simulink model "powertrain"  (R2020b)
settings: Solver=FixedStepAuto  StartTime=0.0  StopTime=t(end)  RelTol=1e-3
PreLoadFcn:
  | C_sc = 1;
StartFcn:
  | C_sc = 1;
values from neighbouring files (symbols this model uses):
  D = 0    [model_fc.m]
  Ts = old_data.Ts    [model_fc.m]
undefined symbols (not defined in the file or in its folder): ANFIS, command, DiscIntNeverNeededParam, ECMS, Flight, in, Ion, Lithium, MPC, out, Tmpc, w
libraries: powerlib x25, neural x25, fuzblock x5, electricdrivelib x3, lib_converters x3, simulink x3, re_lib x1
(part 1 of 8)
PostSaveFcn:
  | C_sc = 1;
settings Model: SimulationMode=accelerator  Creator=maloc  LastModifiedBy=maloc
settings OptimizationCC: DefaultParameterBehavior=Inlined  EnhancedBackFolding=on  PassReuseOutputArgsAs=Individual arguments  ZeroExternalMemoryAtStartup=off  ZeroInternalMemoryAtStartup=off  OptimizeBlockOrder=speed  DifferentSizesBufferReuse=on  OptimizationCustomize=off  EfficientTunableParamExpr=on
settings DebuggingCC: ParameterTunabilityLossMsg=error  SFUnexpectedBacktrackingDiag=warning  SFNoUnconditionalDefaultTransitionDiag=warning
settings SFSimCC: MATLABDynamicMemAlloc=off
settings RTWCC: Description=Embedded Coder  SystemTargetFile=ert.tlc  GenCodeOnly=on  TemplateMakefile=ert_default_tmf  GenerateReport=on  BuildConfiguration=Debug  LaunchReport=on
settings CodeAppCC: ForceParamTrailComments=on  IgnoreCustomStorageClasses=off  OperatorAnnotations=on  SimulinkDataObjDesc=on  SFDataObjDesc=on  InsertBlockDesc=on  EnableCustomComments=on
settings ERTTargetCC: TargetLangStandard=C99 (ISO)  GenerateSampleERTMain=on  InlinedParameterPlacement=NonHierarchical  ERTCustomFileTemplate=example_file_process.tlc

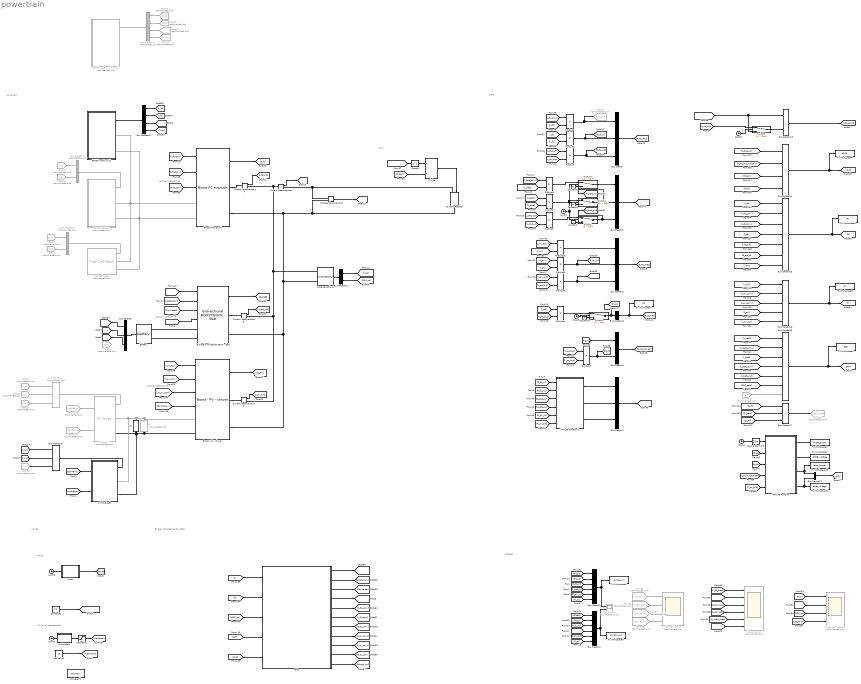
== system powertrain ==
  note: ACTIVE / DESACTIVE
  note: Pload
  note: Data
  note: Powertrain
  note: Energy Management System
  note: SCOPES
  note: Load
  note: Inputs
  note: ACTIVE / DESACTIVE
  note: ACTIVE / DESACTIVE
  note: PV Panel weather data
  Battery : electricdrivelib/Extra Sources/Battery  BatType=Lithium-Ion  ShowTempParam=off  ThermalPreset=no  ShowAgeParam=off  NomV=48  NomQ=15  SOC=80  Batt_Tr=20  PresetModel=on  MaxQ=15  MinV=36  FullV=55.8714  Dis_rate=6.5217  R=0.032  Normal_OP=13.5652  expZone="[51.8585     0.736957]"  current=[2 5 10 40]  Units=Time  Tci=20  NomT=20  T2=-30  MaxQ2=4.8  FullV2=7.1  Normal_OP2=5.655  expZone2="[6.58           1]"  Rca=0.6  ti=2000  Dp=0  Neq0=0  Tsim=Ts  Ta1=25  Qeol=5.4*0.9  Reol=0.013333*1.2  Char_age=[2.3478, 3]  Dis_age=[2.3478, 10]  N1=1500  N2=10500  N3=1000  N4=1400  Ta2=45  N5=950
  Bidirectional BOOST/BUCK - Batt : lib_converters/Bidirectional BOOST//BUCK - Batt  n_buck=0.9  Tr_buck=0.1  damp_buck=0.707  n_boost=0.9  Tr_boost=0.1  damp_boost=0.707  max_curr=[30 -4]  Co=1e-4  CL=C_sc  Li=1e-3  Ts=Ts
  Boost - PV - chsvar : lib_converters/Boost - PV - chsvar  n=0.9  Co=1e-4  CL=C_sc  Li=2e-3  damp=0.707  Tr=0.1  Ts=Ts
  Boost FC avg-swh : lib_converters/Boost FC avg-swh  conv_type=Average model  n=0.9  Co=1e-4  CL=C_sc  Li=2e-3  damp=0.707  Tr=1  Ts=Ts
      link override Discrete PI Controller3: Ts=Ts
  Bus Creator : BusCreator  Inputs=command,in,out
  Bus Creator{1,5,7,17} (4 alike) : BusCreator  Inputs=3
  Bus Creator11 : BusCreator  Inputs=1
  Bus Creator12 : BusCreator  Inputs=2
  Bus Creator13 : BusCreator  Inputs=2
  Bus Creator14 : BusCreator  Inputs=4
  Bus Creator15 : BusCreator  Inputs=7
  Bus Creator16 : BusCreator  Inputs=5
  Bus Creator18 : BusCreator  Inputs=7
  Bus Creator2 : BusCreator  Inputs=6
  Bus Creator3 : BusCreator  Inputs=6
  Bus Creator6 : BusCreator  Inputs=2
  Bus Selector : BusSelector  OutputSignals=SOC (%),Current (A),Voltage (V)
  Bus Selector1 : BusSelector  OutputSignals=Current I,SOC %
  Bus Selector2 : BusSelector  Commented=on  OutputSignals=V_PV,I_PV,Temperature (deg C)
  Bus Selector3 : BusSelector  Commented=on  OutputSignals=Voltage,Current
  Bus Selector4 : BusSelector  Commented=on  OutputSignals=Vout,Ifc
  Bus Selector5 : BusSelector  OutputSignals=V_PV,I_PV,Temperature (deg C)
  Bus Selector6 : BusSelector  OutputSignals=Vout,Ifc,E_act_d,limit
  Bus Selector7 : BusSelector  Commented=on  OutputSignals=Vout,Ifc,E_act_d,limit
  C2 : powerlib/Elements/Series RLC Branch  LConnTagsString=__new0  RConnTagsString=__new0  BranchType=C  Resistance=0.01  Inductance=1e-3  SetiL0=off  InitialCurrent=0  Capacitance=1e-3  Setx0=off  InitialVoltage=0  Measurements=None
  Clock{1..6} (6 alike) : Clock
  Comparison : Scope  Commented=on  NumInputPorts=2
  Constant{,1..3} (4 alike) : Constant  Value=0
  Constant5 : Constant  Value=25
  Constant6 : Constant  Value=72
  Control output : Scope  Commented=on  NumInputPorts=4
  Current Measurement{,2..4} (4 alike) : powerlib/Measurements/Current Measurement  PhasorSimulation=off  OutputType=Complex  PSBequivalent=0
  Divide : Product  Inputs=*/
  EMS : Subsystem  VariantControl=Choice  mask(Energy Management System | Strategy){IO_pv_conv=Yes, IO_fc_conv=Yes, IO_batt_conv=Yes, cont_pv=MPPT, Ts=Ts, ems=EEMS}
      mask prompts: IO_pv_conv "Activate PV converter"; IO_fc_conv "Activate FC converter"; IO_batt_conv "Activate Battery converter"; cont_pv "Control Mode PV converter"; Ts "Sample Time"; ems "Strategy :"
      mask init:
      | SimulinkModel  = [gcs,'/EMS'];
      | SimulinkModel2 = [gcs,'/EMS/Management Variant'];
      | 
      | % if ~exist('Sim_from_m_file','var')
      |     switch ems
      |         case 'None'
      |             disp('No EMS selected')
      |         
      |         case 'CONSTANT'
      |             set_param(SimulinkModel2,'OverrideUsingVariant','CONSTANT');
      | 
      |         case 'SMC'
      |             set_param(SimulinkModel2,'OverrideUsingVariant','SMC');
      | 
      |         case 'FUZZY'
      |             set_param(SimulinkModel2,'OverrideUsingVariant','FUZZY');
      | 
      |         case 'PI'
      |             set_param(SimulinkModel2,'OverrideUsingVariant','PI');
      | 
      |         case 'ECMS'
      |             set_param(SimulinkModel2,'OverrideUsingVariant','ECMS');
      | 
      |         case 'EEMS'
      |             set_param(SimulinkModel2,'OverrideUsingVariant','EEMS');
      | 
      |         case 'D-ECMS'
      |             set_param(SimulinkModel2,'OverrideUsingVariant','D-ECMS');
      |             
      |         case 'MPC-1'
      |         set_param(SimulinkModel2,'OverrideUsingVariant','MPC-1');
      |         
      |         case 'ANFIS'
      |             set_param(SimulinkModel2,'OverrideUsingVariant','ANFIS-ECMS');
      | 
      |         case 'ECAEMS'
      |         set_param(SimulinkModel2,'OverrideUsingVariant','ECAEMS');
      | 
      |     
      |     end
      | % end
      | 
      | switch IO_pv_conv
      |     case 'Yes'
      |         IO_pv_conv_value = 1;
      |     case 'No'
      |         IO_pv_conv_value = 0;
      | end
      | 
      | switch IO_fc_conv
      |     case 'Yes'
      |         IO_fc_conv_value = 1;
      |     case 'No'
      |         IO_fc_conv_value = 0;
      | end
      | 
      | switch IO_batt_conv
      |     case 'Yes'
      |         IO_batt_conv_value = 1;
      |     case 'No'
      |         IO_batt_conv_value = 0;
      | end
      | 
      | switch cont_pv
      |     case 'Auto'
      |         cont_var_pv = 0;
      |     case 'MPPT'
      |         cont_var_pv = 1;
      |     case 'Cascade'
      |         cont_var_pv = 2;
      | end
      mask TypeOptions IO_pv_conv: Yes | No
      mask TypeOptions IO_fc_conv: Yes | No
      mask TypeOptions IO_batt_conv: Yes | No
      mask TypeOptions cont_pv: Auto | MPPT | Cascade
      mask TypeOptions ems: None | CONSTANT | SMC | FUZZY | PI | ECMS | EEMS | D-ECMS | MPC-1 | ANFIS | ECAEMS
  From100 : From  Commented=on  GotoTag=Irradiation
  From102 : From  Commented=on  GotoTag=CellTemp
  From35 : From  Commented=on  GotoTag=Age
  From55 : From  Commented=on  GotoTag=I_fc_conv
  From56 : From  Commented=on  GotoTag=I_batt_conv
  From57 : From  Commented=on  GotoTag=I_pv_conv
  From58 : From  Commented=on  GotoTag=Converter
  Fuel Cell Stack : electricdrivelib/Extra Sources/Fuel Cell Stack  Commented=on  PresetModel=No (User-Defined)  FcType=0  Detailed=Detailed  Eoc=[48,47]  NomVI=[35,32.5]  EndVI=[38,32]  Nc=50  n=50  TOp=55  AirFr=1000  SuppPress=[0.506625,1]  Comp=[99.995,21,1]  SignX=off  SignY=off  FlowRateH2=off  FlowRateAir=off  SystemTemp=off  SystemPH2=off  SystemPAir=off  FCDyn=on  FC_tau=1  Peak_O2=80  V_Under=10
      settings: SourceProductBaseCode=PS
  Goto20 : Goto  Commented=on  GotoTag=V_pv
  Goto21 : Goto  Commented=on  GotoTag=I_pv
  Goto22 : Goto  Commented=on  GotoTag=T_pv
  Goto24 : Goto  Commented=on  GotoTag=V_fc
  Goto28 : Goto  Commented=on  GotoTag=I_fc
  Goto36 : Goto  Commented=on  GotoTag=T_pv
  Goto38 : Goto  Commented=on  GotoTag=Age
  Goto41 : Goto  Commented=on  GotoTag=P_fc_com
  Goto54 : Goto  Commented=on  GotoTag=E_act_d
  Goto55 : Goto  Commented=on  GotoTag=Duty_Cycles  TagVisibility=global
  Goto56 : Goto  Commented=on  GotoTag=V_fc
  Goto6 : Goto  Commented=on  GotoTag=V_fc
  Goto68 : Goto  Commented=on  GotoTag=I_fc
  Goto69 : Goto  Commented=on  GotoTag=limit
  Goto7 : Goto  Commented=on  GotoTag=I_fc
  Important scopes : Scope  Commented=on  NumInputPorts=4
  Load1 : Subsystem  Variant=on  VariantControlMode=label  VariantControl=Choice  LabelModeActiveChoice=Flight-noise  mask{Choice=Flight with noise, CstVal=500, InitVal=500, EndVal=1000, StepTime=10, Scheme1=[0,0,50,500,1000,1250,1250,1000,750,750,750], Break1=[0,2,4,6,8,10,12,14,16,18,20], Scheme2=[0,0,0,1500,1500,1500,1500,1500,1500,1500,1500,1250,1000,1000,1000,1000,1000,1000,1000,1000,1000,1000,1000,1000,1000,1000,1250,1500,1500,1500,1500,1500,1500,1500,1500,1500,1500,0,0,0,0,0], Break2=[0,1.463415e+00,2.926829e+00,4.390244e+00,5.853659e+00,7.317073e+00,8.780488e+00,1.024390e+01,1.170732e+01,1.317073e+01,1.463415e+01,1.609756e+01,1.756098e+01,1.902439e+01,2.048780e+01,2.195122e+01,2.341463e+01,2.487805e+01,2.634146e+01,2.780488e+01,2.926829e+01,3.073171e+01,3.219512e+01,3.365854e+01,3.512195e+01,3.658537e+01,3.804878e+01,3.951220e+01,4.097561e+01,4.243902e+01,4.390244e+01,4.536585e+01,4.682927e+01,4.829268e+01,4.975610e+01,5.121951e+01,5.268293e+01,5.414634e+01,5.560976e+01,5.707317e+01,5.853659e+01,60], Scheme3=[0,0,0,1500,1500,1500,1500,1500,1500,1500,1500,1500,1500,1500,1250,1000,1000,1000,1000,1000,1000], Break3=[0,1,2,3,4,5,6,7,8,9,10,11,12,13,14,15,16,17,18,19,20], Scheme4=w, Break4=t, Scheme5=[0,0,0,1500,1500,1500,1500,1500,1500,1500,1500,1250,1000,1000,1000,1000,1000,1000,1000,1000,1000,1000,1000,1000,1000,1000,1250,1500,1500,1500,1500,1500,1500,1500,1500,1500,1500,1250,1000,1000,1000,1000,1000,1000,1000,1000,1000,1000,1000,1000,1000,1000,1250,1500,1500,1500,1500,1500,1500,1500,1500,1250,1000,1000,1000,1000,1000,1000,1000,1000,1000,1000,1000,1000,1000,1000,1250,1500,1500,1500,1500,1500,1500,1500,1500,1500,1500,1500,1500,1500,1500,1500,1500,1500,1500,1250,1000,1000,1000,1000,1000,1000,1000,1000,1000,1000,1000,1000,1000,1000,1250,1500,1500,1500,1500,1500,1500,1500,1500,1500,1500,1500,1500,1500,1500,1500,1500,1500,1500,1250,1000,1000,1000,1000,1000,1000,1000,1000,1000,1000,1000,1000,1000,1000,1250,1500,1500,1500,1500,1500,1500,1500,1500,1500,1500,0,0,0,0,0], Break5=[0,6.289308e+00,1.257862e+01,1.886792e+01,2.515723e+01,3.144654e+01,3.773585e+01,4.402516e+01,5.031447e+01,5.660377e+01,6.289308e+01,6.918239e+01,7.547170e+01,8.176101e+01,8.805031e+01,9.433962e+01,1.006289e+02,1.069182e+02,1.132075e+02,1.194969e+02,1.257862e+02,1.320755e+02,1.383648e+02,1.446541e+02,1.509434e+02,1.572327e+02,1.635220e+02,1.698113e+02,1.761006e+02,1.823899e+02,1.886792e+02,1.949686e+02,2.012579e+02,2.075472e+02,2.138365e+02,2.201258e+02,2.264151e+02,2.327044e+02,2.389937e+02,2.452830e+02,2.515723e+02,2.578616e+02,2.641509e+02,2.704403e+02,2.767296e+02,2.830189e+02,2.893082e+02,2.955975e+02,3.018868e+02,3.081761e+02,3.144654e+02,3.207547e+02,3.270440e+02,3.333333e+02,3.396226e+02,3.459119e+02,3.522013e+02,3.584906e+02,3.647799e+02,3.710692e+02,3.773585e+02,3.836478e+02,3.899371e+02,3.962264e+02,4.025157e+02,4.088050e+02,4.150943e+02,4.213836e+02,4.276730e+02,4.339623e+02,4.402516e+02,4.465409e+02,4.528302e+02,4.591195e+02,4.654088e+02,4.716981e+02,4.779874e+02,4.842767e+02,4.905660e+02,4.968553e+02,5.031447e+02,5.094340e+02,5.157233e+02,5.220126e+02,5.283019e+02,5.345912e+02,5.408805e+02,5.471698e+02,5.534591e+02,5.597484e+02,5.660377e+02,5.723270e+02,5.786164e+02,5.849057e+02,5.911950e+02,5.974843e+02,6.037736e+02,6.100629e+02,6.163522e+02,6.226415e+02,6.289308e+02,6.352201e+02,6.415094e+02,6.477987e+02,6.540881e+02,6.603774e+02,6.666667e+02,6.729560e+02,6.792453e+02,6.855346e+02,6.918239e+02,6.981132e+02,7.044025e+02,7.106918e+02,7.169811e+02,7.232704e+02,7.295597e+02,7.358491e+02,7.421384e+02,7.484277e+02,7.547170e+02,7.610063e+02,7.672956e+02,7.735849e+02,7.798742e+02,7.861635e+02,7.924528e+02,7.987421e+02,8.050314e+02,8.113208e+02,8.176101e+02,8.238994e+02,8.301887e+02,8.364780e+02,8.427673e+02,8.490566e+02,8.553459e+02,8.616352e+02,8.679245e+02,8.742138e+02,8.805031e+02,8.867925e+02,8.930818e+02,8.993711e+02,9.056604e+02,9.119497e+02,9.182390e+02,9.245283e+02,9.308176e+02,9.371069e+02,9.433962e+02,9.496855e+02,9.559748e+02,9.622642e+02,9.685535e+02,9.748428e+02,9.811321e+02,9.874214e+02,9.937107e+02,1000]}
      mask prompts: Choice "Load"; CstVal "Constant Load value (Power)"; InitVal "Init value (Power)"; EndVal "End Value (Power)"; StepTime "Step time"; Scheme1 "Scheme data (Power)"; Break1 "Breakpoints"; Scheme2 "Scheme data (Power)"; Break2 "Breakpoints"; Scheme3 "Scheme data (Power)"; Break3 "Breakpoints"; Scheme4 "Scheme data (Power)"; Break4 "Breakpoints"; Scheme5 "Scheme data (Power)"; Break5 "Breakpoints"
      mask help: Power in W
      mask init:
      | %Choose between control type
      | SimulinkModel  = [gcb,'/'];
      | 
      | switch Choice
      |     case 'Constant'
      |         set_param(gcb,'OverrideUsingVariant','Constant');
      |         
      |     case 'Step'
      |         set_param(gcb,'OverrideUsingVariant','Step');
      |         
      |     case 'Flight scheme 1'
      |         set_param(gcb,'OverrideUsingVariant','Flight-1');
      |         
      |     case 'Flight scheme 2'
      |         set_param(gcb,'OverrideUsingVariant','Flight-2');
      |         
      |     case 'Flight scheme 3'
      |         set_param(gcb,'OverrideUsingVariant','Flight-3');
      |         
      |     case 'Flight with noise'
      |         set_param(gcb,'OverrideUsingVariant','Flight-noise');
      |         
      |     case 'Real flight'
      |         set_param(gcb,'OverrideUsingVariant','Flight-real');
      | end
      | 
      | %Flight scheme 1
      | %Flight scheme 2
      mask TypeOptions Choice: Constant | Step | Flight scheme 1 | Flight scheme 2 | Flight scheme 3 | Flight with noise | Real flight
      mask DialogControl Container3 Prompt: Constant
      mask DialogControl Container10 Prompt: Step Values
      mask DialogControl Container5 Prompt: Flight Scheme 1
      mask DialogControl Container6 Prompt: Flight Scheme 2
      mask DialogControl Container7 Prompt: Flight Scheme 3
      mask DialogControl Container8 Prompt: Flight Scheme with noise
      mask DialogControl Container9 Prompt: Real Flight Scheme
  MATLAB Function : MATLAB Function  TreatAsAtomicUnit=on
  MATLAB Function1 : MATLAB Function  TreatAsAtomicUnit=on
  PEMFC matfunc : Subsystem  Commented=on  mask{P_H2=0.5, P_O2=1, T=313.15, W=14, tm=1.27e-4, Nfc=50, Rohm=0.061871, Ts=1e-4, fc_tau=1}
      mask prompts: P_H2 "Hydrogen pressure (atm)"; P_O2 "Oxygen pressure (atm)"; T "Temperature (K)"; W "Water Content"; tm "Thickness of the membrane (m)"; Nfc "Number of cells"; Rohm "Fuel cell resistance"; Ts "Sample time (s)"; fc_tau "Dynamic response of the FC (s)"
      mask init:
      | tau = fc_tau / 5;
  PEMFC matfunc V2 : Subsystem  mask{P_H2=0.5, P_O2=1, T=313.15, W=14, tm=1.27e-4, Nfc=50, Rohm=0.061871, Ts=Ts, fc_tau=1}
      mask prompts: P_H2 "Hydrogen pressure (atm)"; P_O2 "Oxygen pressure (atm)"; T "Temperature (K)"; W "Water Content"; tm "Thickness of the membrane (m)"; Nfc "Number of cells"; Rohm "Fuel cell resistance"; Ts "Sample time (s)"; fc_tau "Dynamic response of the FC (s)"
      mask init:
      | tau = fc_tau / 5;
  PEMFC matfunc V3 - multi : Subsystem  Commented=on  mask{P_H2=0.5, P_O2=1, T=313.15, W=14, tm=1.27e-4, Nfc=50, Rohm=0.061871, Ts=Ts, fc_tau=1}
      mask prompts: P_H2 "Hydrogen pressure (atm)"; P_O2 "Oxygen pressure (atm)"; T "Temperature (K)"; W "Water Content"; tm "Thickness of the membrane (m)"; Nfc "Number of cells"; Rohm "Fuel cell resistance"; Ts "Sample time (s)"; fc_tau "Dynamic response of the FC (s)"
      mask init:
      | tau = fc_tau / 5;
  PV MODULE1 : Subsystem  mask{Npar=1, Nser=1, Ncell=72, Pm=0, Voc=44.5, Isc=5.54, Vmpp=37.2, Impp=4.97, beta_Voc_pc=-0.34, alpha_Isc_pc=-0.017, beta_Voc=0, alpha_Isc=0, IL=5.55564, I0=2.39143e-10, df=0.96618, Rsh=113.762, Rs=0.32122, Ts=Ts}
      mask prompts: Npar "Parallel connected modules"; Nser "Series connected modules"; Ncell "Number of cells per module"; Pm "Maxium Power (W)"; Voc "Open circuit voltage Voc (V)"; Isc "Short-circuit current Isc (A)"; Vmpp "Voltage at MPP (V)"; Impp "Current at MPP (A)"; beta_Voc_pc "Temperature coefficient of Voc (%/deg.C"; alpha_Isc_pc "Temperature coefficient of Isc (%/deg.C)"; beta_Voc "Temperature coefficient of Voc (V/deg.C)"; alpha_Isc "Temperature coefficient of Isc (A/deg.C)"; IL "Light-generated current IL (A)"; I0 "Diode saturation current I0 (A)"; df "Diode ideality factor"; Rsh "Shunt resistance Rsh (ohms)"; Rs "Series resistance Rs (ohms)"; Ts "Sample time (s)"
      mask init:
      | if alpha_Isc ~= 0
      |     alpha = alpha_Isc;
      | else 
      |     alpha = alpha_Isc_pc * Isc/100;
      | end
      mask DialogControl Container5 Prompt: Module data
      mask DialogControl Container3 Prompt: Data from data sheet
      mask DialogControl Container6 Prompt: Data from NREL
  Power scopes : Scope  Commented=on  NumInputPorts=6
  Product{,1..10} (11 alike) : Product
  R : powerlib/Elements/Series RLC Branch  Commented=on  LConnTagsString=__new0  RConnTagsString=__new0  BranchType=R  Resistance=1e6  Inductance=1e-3  SetiL0=off  InitialCurrent=0  Capacitance=1e-6  Setx0=off  InitialVoltage=0  Measurements=None
  Saturation : Saturate  UpperLimit=1000  LowerLimit=0
  Sopray 1 : re_lib/Solar/PV Array  Commented=on  Npar=1  Nser=1  PlotType=array @ 1000 W/m2 & specified temperatures  S_vec="[ 1000  500  100 ]"  Temp_C_vec="[ 45 25  ]"  ModuleName=User-defined  PlotWhenSelected=off  Pm=184.884  Ncell=72  Voc=44.5  Isc=5.54  Vm=37.2  Im=4.97  beta_Voc_pc=-0.34  alpha_Isc_pc=-0.017  beta_Voc=-0.1513  alpha_Isc=-0.0009418  IL=5.558  I0=7.9256e-11  nI=0.96618  Rsh=110.2917  Rs=0.35764  RobustModel=off  RobustCellTemperature=313.3991  BAL=on  Tc=1e-6  Tfilter=5e-5
  Square : Math  Operator=square  SaturateOnIntegerOverflow=on
  Subsystem : Subsystem  Variant=on  VariantControlMode=label  VariantControl=Choice  LabelModeActiveChoice=Constant  mask{Choice=Constant, irradiance_const=800, irradiance1=[9.978198e-01,9.978198e-01,9.978198e-01], break1=[0,30,60], irradiance_step_init=1000, irradiance_step_end=500, break_step=5}
      mask prompts: Choice "Choose the model"; irradiance_const "Irradiance (W/m2)"; irradiance1 "Irradiance (W/m2)"; break1 "Time (s)"; irradiance_step_init "Irradiance init (W/m2)"; irradiance_step_end "Irradiance end (W/m2)"; break_step "Step Time (s)"
      mask init:
      | %Choose between control type
      | SimulinkModel  = [gcb,'/'];
      | 
      | switch Choice
      |     case 'Constant'
      |         set_param(gcb,'OverrideUsingVariant','Constant');
      |         
      |     case 'Step'
      |         set_param(gcb,'OverrideUsingVariant','Step');
      |         
      |     case 'Model-1'
      |         set_param(gcb,'OverrideUsingVariant','Model1');
      | end
      mask TypeOptions Choice: Constant | Step | Model-1
      mask DialogControl Container7 Prompt: Choose type irradiance model
      mask DialogControl Container5 Prompt: Constant
      mask DialogControl Container3 Prompt: Irradiance model 1
      mask DialogControl Container4 Prompt: Irradiance step
  Supercapacitor1 : electricdrivelib/Extra Sources/Supercapacitor  C=1  Rdc=150e-3  Voltage=72  Ns=50  Np=1  Vinit=72  Temp=25  PresetModel=on  EstParam=off  Nc=1  r=1e-9  epsilon=6.0208e-10  Ich=10  Vstern="[0.161  2.7  7.8]"  Self_dis=on  Ioc=10  Vself="[48  47.8  47.06  44.65]"  demandeplot=off  I="[10  20 100  500]"  Units=sec  Vmax=0  If=0  deltaV=0.3  alpha=0.3  sec=0
      settings: SourceProductBaseCode=PS
  Switch{1..2,4..6} (5 alike) : Switch  Criteria=u2 > Threshold  Threshold=2e-4
  To Workspace1 : ToWorkspace  VariableName=RMSE_power  SaveFormat=Timeseries  SampleTime=-1
  To Workspace11 : ToWorkspace  VariableName=error_power  SaveFormat=Timeseries  SampleTime=-1
  To Workspace12 : ToWorkspace  VariableName=error_voltage  SaveFormat=Timeseries  SampleTime=-1
  To Workspace2 : ToWorkspace  VariableName=RMSE_voltage  SaveFormat=Timeseries  SampleTime=-1
  To Workspace3 : ToWorkspace  VariableName=FC  SaveFormat=Structure  SampleTime=-1
      settings: Save2DSignal=2-D array (concatenate along first dimension)
  To Workspace4 : ToWorkspace  VariableName=Batt  SaveFormat=Structure  SampleTime=-1
      settings: Save2DSignal=2-D array (concatenate along first dimension)
  To Workspace5 : ToWorkspace  VariableName=LOAD  SaveFormat=Structure  SampleTime=-1
      settings: Save2DSignal=2-D array (concatenate along first dimension)
  To Workspace6 : ToWorkspace  VariableName=PV  SaveFormat=Structure  SampleTime=-1
      settings: Save2DSignal=2-D array (concatenate along first dimension)
  To Workspace7 : ToWorkspace  VariableName=SC  SaveFormat=Structure  SampleTime=Ts
      settings: Save2DSignal=2-D array (concatenate along first dimension)
  To Workspace8 : ToWorkspace  VariableName=compar_out  SaveFormat=Structure  SampleTime=Ts
      settings: Save2DSignal=2-D array (concatenate along first dimension)
  To Workspace9 : ToWorkspace  VariableName=compar_in  SaveFormat=Structure  SampleTime=Ts
      settings: Save2DSignal=2-D array (concatenate along first dimension)
  Variable Resistor : powerlib/Elements/Variable Resistor  Rabsmin=1e-3
      settings: SourceProductBaseCode=PS
  Voltage Measurement : powerlib/Measurements/Voltage Measurement  PhasorSimulation=off  OutputType=Complex  PSBequivalent=0
  Zero-Order Hold : ZeroOrderHold  SampleTime=Ts
  powergui1 : powerlib/powergui  Priority=1  SimulationMode=Discrete  SampleTime=Ts  frequency=60  Iterations=50  frequencyindice=0  Pbase=100e6  ErrMax=1e-4  UnitsV=kV  UnitsW=MW  buscounter=0  FunctionMessages=off  echomessages=off  EnableUseOfTLC=off  CurrentSourceSwitches=off  DisableSnubberDevices=off  DisableRonSwitches=off  DisableVfSwitches=off  DisplayEquations=off  AutomaticDiscreteSolvers=off  SolverType=Tustin/Backward Euler (TBE)  Interpol=off  ExternalGateDelay=off  methode=off  Ts=100  x0status=blocks  SPID=on  SwTol=0  HookPort=off  NonlinearTolerance=1e-4  nMaxIteration=100  ContinueOnMaxIteration=off  RestoreLinks=warning  ResistiveCurrentMeasurement=off  Frange=[0:2:500]  Ylog=off  Xlog=on  ShowGrid=off  save=off  variable=ZData  structure=0  ZoomFFT=off  StartTime=0.0  cycles=1  DisplayStyle=1  fundamental=60  FreqAxis=off  MaxFrequency=1000  frequencyindicesteady=1  RmsSteady=1  display=off
  tag scope: BATT=global, FC=global, LOAD=global, PV=global, V_dc_comp=global, error=global
  wires:
  Constant6/1 -> [V_dc_bus_wanted]  "Vbus_required"
  [V_batt_conv] -> Bidirectional BOOST/BUCK - Batt/1
  [I_batt_conv] -> Bidirectional BOOST/BUCK - Batt/2
  Battery/1 -> Bus Selector/1  "BATT"
  Current Measurement4/1 -> [I_fc_out]  "Ifc_output"
  Current Measurement3/1 -> [I_batt_out]  "Ibatt_output"
  Supercapacitor1/1 -> Bus Selector1/1
  Voltage Measurement/1 -> [V_dc_bus]  "Vbus_real"
  Bus Creator/1 -> [P_FC_mes]  "FC power"
  Product2/1 -> [P_fc_in], Bus Creator/2  "in"
  Product/1 -> [P_fc_out], Bus Creator/3  "out"
  Product4/1 -> Switch5/1  "out"
  Bus Selector1/1 -> [I_sc]  "<Current I>"
  Current Measurement/1 -> [I_dc_bus]  "OUTPUT"
  [IO_pv_conv] -> Boost - PV - chsvar/3
  Current Measurement2/1 -> [I_pv_out]  "Ibatt_output"
  Sopray 1/1 -> Bus Selector2/1
  Bus Selector2/1 -> Goto20/1  "<V_PV>"
  Bus Selector2/2 -> Goto21/1  "<I_PV>"
  Bus Selector2/3 -> Goto22/1  "<Temperature (deg C)>"
  [V_fc] -> Product2/2
  [I_fc] -> Product2/1
  [I_fc_out] -> Product/1
  [V_dc_bus] -> Product/2
  [V_dc_bus] -> Product1/2
  [I_batt_out] -> Product1/1
  [I_batt] -> Product3/1
  [V_batt] -> Product3/2
  Product1/1 -> Switch2/1  "out"
  Product3/1 -> Switch1/1  "in"
  Bus Creator1/1 -> [P_batt_mes]  "BATT power"
  Bus Creator5/1 -> [P_PV_mes]  "PV power"
  Product6/1 -> [P_pv_in], Bus Creator5/2  "in"
  Product5/1 -> [P_pv_out], Bus Creator5/3  "out"
  [V_pv] -> Product6/2
  [I_pv] -> Product6/1
  [I_pv_out] -> Product5/1
  [V_dc_bus] -> Product5/2
  [I_sc] -> Product4/1
  [V_dc_bus] -> Product4/2
  [I_dc_bus] -> Product7/1
  [V_dc_bus] -> Product7/2
  [V_dc_bus_wanted] -> Square/1
  Square/1 -> Divide/1
  [Pload] -> Divide/2
  Divide/1 -> Variable Resistor/1
  From102/1 -> Sopray 1/2
  [I_pv_conv] -> Boost - PV - chsvar/2
  [V_pv_conv] -> Boost - PV - chsvar/1
  Product7/1 -> [Pout], Bus Creator6/2  "real"
  [Pload] -> Bus Creator6/1  "required"
  Bus Creator6/1 -> [P_Load_mes]  "Load power"
  [I_fc_conv] -> Product8/1
  [V_fc] -> Product8/2
  Product8/1 -> Goto41/1, Bus Creator/1  "command"
  [V_batt] -> Product9/2
  [I_batt_conv] -> Product9/1
  Product9/1 -> Switch4/1  "command"
  [I_pv_conv] -> Product10/1
  Product10/1 -> Bus Creator5/1  "command"
  [V_pv] -> Product10/2
  [SOC_batt] -> Important scopes/2  "Batt SOC"
  Bus Selector1/2 -> [SOC_sc]  "<SOC %>"
  [SOC_sc] -> Important scopes/3  "SC SOC"
  [Converter] -> Bidirectional BOOST/BUCK - Batt/3
  From55/1 -> Control output/1  "FC current"
  From56/1 -> Control output/2  "Batt current"
  From57/1 -> Control output/3  "PV current"
  From58/1 -> Control output/4  "converter"
  Subsystem/1(Out1) -> Saturation/1
  Clock1/1 -> Switch4/2, Switch1/2, Switch2/2
  Switch1/1 -> [P_batt_in], Bus Creator1/2  "in"
  Switch2/1 -> [P_batt_out], Bus Creator1/3  "out"
  Bus Selector4/1 -> Goto24/1  "<Vout>"
  Bus Selector4/2 -> Goto28/1  "<Ifc>"
  PEMFC matfunc/1(output) -> Bus Selector4/1
  MATLAB Function1/1(FC) -> Bus Creator7/1  "FC"
  MATLAB Function1/2(BATT) -> Bus Creator7/2  "BATT"
  MATLAB Function1/3(PV) -> Bus Creator7/3  "PV"
  Bus Creator7/1 -> [Efficiencies]  "Efficiency"
  Bus Creator11/1 -> To Workspace7/1, [P_sc_mes]  "SC power"
  [P_FC_mes] -> Power scopes/1  "FC"
  [P_batt_mes] -> Power scopes/2  "Batt"
  [P_PV_mes] -> Power scopes/3  "PV"
  [P_sc_mes] -> Power scopes/4  "SC"
  [P_Load_mes] -> Power scopes/5  "Load"
  [Efficiencies] -> Power scopes/6  "Efficiency"
  [error] -> Important scopes/1  "errors (%)"
  Bus Creator12/1 -> [error]  "error (%)"
  Switch4/1 -> Bus Creator1/1  "command"
  Clock5/1 -> Switch5/2
  Switch5/1 -> [P_sc], Bus Creator11/1  "out"
  [V_dc_bus] -> Switch6/1  "real"
  Bus Creator13/1 -> [V_dc_comp]  "V dc bus"
  [V_dc_comp] -> Important scopes/4  "DC bus voltage"
  Saturation/1 -> [Irradiation]  "radiation"
  From100/1 -> Sopray 1/1
  Constant5/1 -> [CellTemp]
  [V_dc_bus] -> Bus Creator14/1  "Vbus real"
  [V_dc_bus_wanted] -> Bus Creator14/2  "Vbus required"
  [Pload] -> Bus Creator14/3  "Pload required"
  [V_fc] -> Bus Creator15/1  "Vfc"
  [I_fc] -> Bus Creator15/4  "Ifc"
  [I_fc_out] -> Bus Creator15/5  "Ifc out"
  [V_pv] -> Bus Creator16/1
  [I_pv_conv] -> Bus Creator16/3
  [I_pv] -> Bus Creator16/4
  [I_pv_out] -> Bus Creator16/5
  Bus Creator14/1 -> To Workspace5/1, [LOAD]  "LOAD"
  Bus Creator16/1 -> To Workspace6/1, [PV]  "PV"
  Bus Creator15/1 -> To Workspace3/1, [FC]  "FC"
  [LOAD] -> EMS/5(LOAD)
  [FC] -> EMS/2(FC)
  [PV] -> EMS/1(PV)
  Clock6/1 -> Load1/1(In1)
  Load1/1(Out1) -> [Pload]
  Bidirectional BOOST/BUCK - Batt/1 -> [D_batt]
  Bus Creator17/1 -> Goto55/1  "Duty Cycles"
  [D_fc] -> Bus Creator17/1  "Dfc"
  [D_batt] -> Bus Creator17/2  "Dbatt"
  [D_PV] -> Bus Creator17/3  "Dpv"
  [Control_pv] -> Boost - PV - chsvar/4
  Boost - PV - chsvar/1 -> [D_PV]
  [Pout] -> Bus Creator14/4  "Pload real"
  [SOC_sc] -> EMS/3(SC)
  [BATT] -> EMS/4(BATT)
  [I_fc_conv] -> Bus Creator15/3  "Ifc conv"
  EMS/1(Vbatt_conv) -> [V_batt_conv]
  EMS/2(Ibatt_conv) -> [I_batt_conv]
  EMS/3(batt converter mode) -> [Converter]
  EMS/5(Vfc_conv) -> [V_fc_conv]
  EMS/6(Ifc_conv) -> [I_fc_conv]
  EMS/7(I/O fc conv) -> [IO_fc_conv]
  EMS/8(Vpv_conv) -> [V_pv_conv]
  EMS/9(Ipv_conv) -> [I_pv_conv]
  EMS/10(I/O pv conv) -> [IO_pv_conv]
  EMS/11(PV control mode) -> [Control_pv]
  [IO_batt_conv] -> Bidirectional BOOST/BUCK - Batt/4
  EMS/4(I/O batt conv) -> [IO_batt_conv]
  Bus Selector3/2 -> Goto7/1  "<Current>"
  Bus Selector3/1 -> Goto6/1  "<Voltage>"
  Fuel Cell Stack/1 -> Bus Selector3/1
  Zero-Order Hold/1 -> MATLAB Function/1(time)
  Clock2/1 -> Zero-Order Hold/1
  MATLAB Function/3(error_power) -> Bus Creator12/1, To Workspace11/1
  MATLAB Function/4(error_voltage) -> Bus Creator12/2, To Workspace12/1
  [V_dc_bus_wanted] -> MATLAB Function/4(Vbus_required)
  [V_dc_bus] -> MATLAB Function/5(Vbus_real)
  [Pout] -> MATLAB Function/3(Preal)
  [Pload] -> MATLAB Function/2(Prequired)
  MATLAB Function/1(ep) -> To Workspace1/1
  MATLAB Function/2(ev) -> To Workspace2/1
  [P_fc_in] -> MATLAB Function1/1(Pfc_in)
  [P_fc_out] -> MATLAB Function1/2(Pfc_out)
  [P_pv_in] -> MATLAB Function1/5(Ppv_in)
  [P_pv_out] -> MATLAB Function1/6(Ppv_out)
  [P_batt_out] -> MATLAB Function1/4(Pbatt_out)
  [P_batt_in] -> MATLAB Function1/3(Pbatt_in)
  Bus Creator18/1 -> To Workspace4/1, [BATT]  "BATT"
  [I_batt_out] -> Bus Creator18/5
  [V_batt] -> Bus Creator18/1
  [I_batt] -> Bus Creator18/3
  [I_batt_conv] -> Bus Creator18/4
  [SOC_batt] -> Bus Creator18/6
  [V_dc_bus_wanted] -> Bus Creator13/1, Switch6/3  "wanted"
  Clock3/1 -> Switch6/2
  Switch6/1 -> Bus Creator13/2  "real"
  Constant/1 -> Switch2/3
  Constant1/1 -> Switch1/3
  Constant2/1 -> Switch4/3
  Constant3/1 -> Switch5/3
  [IO_fc_conv] -> Boost FC avg-swh/3
  [I_fc_conv] -> Boost FC avg-swh/2
  [V_fc_conv] -> Boost FC avg-swh/1
  Boost FC avg-swh/1 -> [D_fc]
  Clock4/1 -> Subsystem/1(In1)
  [CellTemp] -> PV MODULE1/1(TempCell_C)
  [Irradiation] -> PV MODULE1/2(Irradiance)
  Bus Selector5/2 -> [I_pv]  "<I_PV>"
  Bus Selector5/1 -> [V_pv]  "<V_PV>"
  PV MODULE1/1(data) -> Bus Selector5/1
  Bus Selector5/3 -> Goto36/1  "<Temperature (deg C)>"
  Bus Creator2/1 -> To Workspace9/1, Comparison/1  "compare_power_in"
  [P_fc_in] -> Bus Creator2/3  "Pfc in"
  [P_batt_in] -> Bus Creator2/4  "P batt in"
  [P_pv_in] -> Bus Creator2/5  "P pv in"
  [P_sc] -> Bus Creator2/6  "P sc"
  [P_sc] -> Bus Creator3/6  "P sc"
  [P_pv_out] -> Bus Creator3/5  "P pv out"
  [P_batt_out] -> Bus Creator3/4  "P batt out"
  [P_fc_out] -> Bus Creator3/3  "P fc out"
  Bus Creator3/1 -> To Workspace8/1, Comparison/2  "compare_power_out"
  [Pout] -> Bus Creator2/2  "Pout real"
  [Pload] -> Bus Creator2/1  "Pout required"
  [Pload] -> Bus Creator3/1  "P out required"
  [Pout] -> Bus Creator3/2  "P out real"
  From35/1 -> Bus Creator18/7
  [V_batt_conv] -> Bus Creator18/2
  [V_pv_conv] -> Bus Creator16/2
  [V_fc_conv] -> Bus Creator15/2
  PEMFC matfunc V2/1(output) -> Bus Selector6/1
  Bus Selector6/1 -> [V_fc]  "<Vout>"
  Bus Selector6/2 -> [I_fc]  "<Ifc>"
  Bus Selector/1 -> [SOC_batt]  "<SOC (%)>"
  Bus Selector/2 -> [I_batt]  "<Current (A)>"
  Bus Selector/3 -> [V_batt]  "<Voltage (V)>"
  ? -> Goto38/1  "<Age (Equivalent Full cycles)>"
  Bus Selector6/3 -> [E_act_d]  "<E_act_d>"
  Bus Selector6/4 -> [limit]  "<limit>"
  [E_act_d] -> Bus Creator15/6
  [limit] -> Bus Creator15/7
  Bus Selector7/4 -> Goto69/1  "<limit>"
  Bus Selector7/3 -> Goto54/1  "<E_act_d>"
  Bus Selector7/2 -> Goto68/1  "<Ifc>"
  Bus Selector7/1 -> Goto56/1  "<Vout>"
  PEMFC matfunc V3 - multi/1(output) -> Bus Selector7/1
  connections:
  Current Measurement/RConn1 -- Variable Resistor/LConn1 -- Voltage Measurement/LConn1
  Voltage Measurement/LConn2 -- Variable Resistor/RConn1 -- Boost - PV - chsvar/RConn2 -- Bidirectional BOOST/BUCK - Batt/RConn2 -- Supercapacitor1/LConn2 -- Boost FC avg-swh/RConn2
  Current Measurement/LConn1 -- Current Measurement4/RConn1 -- Current Measurement2/RConn1 -- Current Measurement3/RConn1 -- Supercapacitor1/LConn1
  Bidirectional BOOST/BUCK - Batt/LConn2 -- Battery/LConn2
  Bidirectional BOOST/BUCK - Batt/LConn1 -- Battery/LConn1
  Bidirectional BOOST/BUCK - Batt/RConn1 -- Current Measurement3/LConn1
  Boost FC avg-swh/RConn1 -- Current Measurement4/LConn1
  C2/RConn1 -- R/RConn1 -- Boost - PV - chsvar/LConn2 -- Sopray 1/RConn2 -- PV MODULE1/RConn2
  Boost - PV - chsvar/RConn1 -- Current Measurement2/LConn1
  Sopray 1/RConn1 -- PV MODULE1/RConn1 -- Boost - PV - chsvar/LConn1 -- R/LConn1 -- C2/LConn1
  PEMFC matfunc/RConn1 -- Boost FC avg-swh/LConn1 -- PEMFC matfunc V2/RConn1 -- Fuel Cell Stack/RConn1
  PEMFC matfunc/RConn2 -- PEMFC matfunc V2/RConn2 -- Boost FC avg-swh/LConn2 -- Fuel Cell Stack/RConn2

== system powertrain/EMS ==
  PV : Inport
  FC : Inport  Port=2
  SC : Inport  Port=3
  BATT : Inport  Port=4
  LOAD : Inport  Port=5
  Management Variant : Subsystem  Variant=on  VariantControlMode=label  VariantControl=Choice  LabelModeActiveChoice=EEMS
  Vbatt_conv : Outport
  Ibatt_conv : Outport  Port=2
  batt converter mode : Outport  Port=3
  I/O batt conv : Outport  Port=4
  Vfc_conv : Outport  Port=5
  Ifc_conv : Outport  Port=6
  I/O fc conv : Outport  Port=7
  Vpv_conv : Outport  Port=8
  Ipv_conv : Outport  Port=9
  I/O pv conv : Outport  Port=10
  PV control mode : Outport  Port=11
  wires:
  FC/1 -> Management Variant/2(FC)
  PV/1 -> Management Variant/1(PV)
  Management Variant/2(Ibatt_conv) -> Ibatt_conv/1
  SC/1 -> Management Variant/3(SC)
  BATT/1 -> Management Variant/4(BATT)
  Management Variant/5(Vfc_conv) -> Vfc_conv/1
  LOAD/1 -> Management Variant/5(LOAD)
  Management Variant/1(Vbatt_conv) -> Vbatt_conv/1
  Management Variant/6(Ifc_conv) -> Ifc_conv/1
  Management Variant/7(I/O fc conv) -> I/O fc conv/1
  Management Variant/8(Vpv_conv) -> Vpv_conv/1
  Management Variant/9(Ipv_conv) -> Ipv_conv/1
  Management Variant/10(I/O pv conv) -> I/O pv conv/1
  Management Variant/3(batt converter mode) -> batt converter mode/1
  Management Variant/11(PV control mode) -> PV control mode/1
  Management Variant/4(I/O batt conv) -> I/O batt conv/1

== system powertrain/Load1 ==
  In1 : Inport
  Constant : Subsystem  VariantControl=Constant
  Flight-1 : Subsystem  VariantControl=Flight-1
  Flight-2 : Subsystem  VariantControl=Flight-2
  Flight-3 : Subsystem  VariantControl=Flight-3
  Flight-noise : Subsystem  VariantControl=Flight-noise
  Flight-real : Subsystem  VariantControl=Flight-real
  Step : Subsystem  VariantControl=Step
  Out1 : Outport

== system powertrain/PEMFC matfunc ==
  Bus Creator : BusCreator  Inputs=10
  Constant : Constant  Value=inf
  Controlled Voltage Source : powerlib/Electrical Sources/Controlled Voltage Source  Initialize=on  Source_Type=AC  Amplitude=0  Phase=0  Frequency=0  Measurements=None
  Current Measurement : powerlib/Measurements/Current Measurement  PhasorSimulation=off  OutputType=Complex  PSBequivalent=0
  Diode2 : powerlib/Power Electronics/Diode  Ron=Rohm  Lon=0  Vf=0  IC=0  UseSnubber=off  Rs=1e4  Cs=inf  Measurements=off
  From9 : From  Commented=on  GotoTag=E
  MATLAB Function : MATLAB Function  TreatAsAtomicUnit=on
  Nfc : Constant  Value=Nfc
  Nfc1 : Constant  Value=Nfc
  P_H1 : Constant  Value=P_H2
  P_O1 : Constant  Value=P_O2
  Product : Product
  Product1 : Product
  Product2 : Product
  Saturation Dynamic : simulink/Discontinuities/Saturation Dynamic  OutMin=[]  OutMax=[]  OutDataTypeStr=Inherit: Same as second input  OutDataType=fixdt(1, 16)  OutScaling=2^-10  DoSatur=off
  Sum : Sum  Inputs=|-+
  Sum1 : Sum  Inputs=+++
  T1 : Constant  Value=T
  Transfer Fcn2 : TransferFcn  Denominator=[tau 1]
  Unit Delay : UnitDelay  SampleTime=Ts  HasFrameUpgradeWarning=on
  Unit Delay1 : UnitDelay  SampleTime=Ts  HasFrameUpgradeWarning=on
  Voltage Measurement : powerlib/Measurements/Voltage Measurement  PhasorSimulation=off  OutputType=Complex  PSBequivalent=0
  W1 : Constant  Value=W
  tm1 : Constant  Value=tm
  + : PMIOPort  Tag=PMCPort  Side=Right
  - : PMIOPort  Tag=PMCPort  Port=2  Side=Right
  output : Outport  VectorParamsAs1DForOutWhenUnconnected=off
  wires:
  P_H1/1 -> MATLAB Function/2(P_H2)
  P_O1/1 -> MATLAB Function/3(P_O2)
  T1/1 -> MATLAB Function/4(T)
  W1/1 -> MATLAB Function/5(Water_content)
  tm1/1 -> MATLAB Function/6(delta_m)
  Nfc/1 -> MATLAB Function/7(Nfc)
  Unit Delay/1 -> MATLAB Function/1(Ifc)  "Current"
  MATLAB Function/2(E_Ner) -> [E_ner]
  MATLAB Function/3(E_act) -> [E_act]
  MATLAB Function/4(E_ohm) -> [E_ohm]
  MATLAB Function/5(E_con) -> [E_con]
  MATLAB Function/1(E) -> [E]
  [Ifc] -> Unit Delay/1
  [E] -> Bus Creator/1  "E"
  [E_ner] -> Bus Creator/2  "E_ner"
  [E_act] -> Bus Creator/3  "E_act"
  [E_ohm] -> Bus Creator/4  "E_ohm"
  [Ifc] -> Product/1, Bus Creator/6  "Ifc"
  [Vout] -> Product/2, Bus Creator/7  "Vout"
  [E_con] -> Bus Creator/5  "E_con"
  Product/1 -> Bus Creator/8  "Pout"
  Current Measurement/1 -> [Ifc]  "Current"
  Voltage Measurement/1 -> [Vout]  "Voltage"
  MATLAB Function/6(U_H2) -> [U_H2]
  MATLAB Function/7(U_O2) -> [U_O2]
  [U_H2] -> Bus Creator/9
  [U_O2] -> Bus Creator/10
  Bus Creator/1 -> output/1
  MATLAB Function/8(Rohm) -> [Rohm]
  Sum1/1 -> Product1/1
  [E_ohm] -> Sum1/2
  Nfc1/1 -> Product1/2
  [E_ner] -> Sum1/1
  [Ifc] -> Unit Delay1/1
  Unit Delay1/1 -> Product2/2  "Current"
  Product1/1 -> Saturation Dynamic/2
  Product2/1 -> Saturation Dynamic/3
  [Rohm] -> Product2/1
  Constant/1 -> Saturation Dynamic/1
  Sum/1 -> Transfer Fcn2/1  "Vact"
  [E_act] -> Sum/2
  Saturation Dynamic/1 -> Controlled Voltage Source/1
  [E_con] -> Sum/1
  Transfer Fcn2/1 -> Sum1/3  "Vact"
  connections:
  -/RConn1 -- Voltage Measurement/LConn2 -- Controlled Voltage Source/LConn1
  +/RConn1 -- Voltage Measurement/LConn1 -- Current Measurement/RConn1
  Diode2/RConn1 -- Current Measurement/LConn1
  Diode2/LConn1 -- Controlled Voltage Source/RConn1

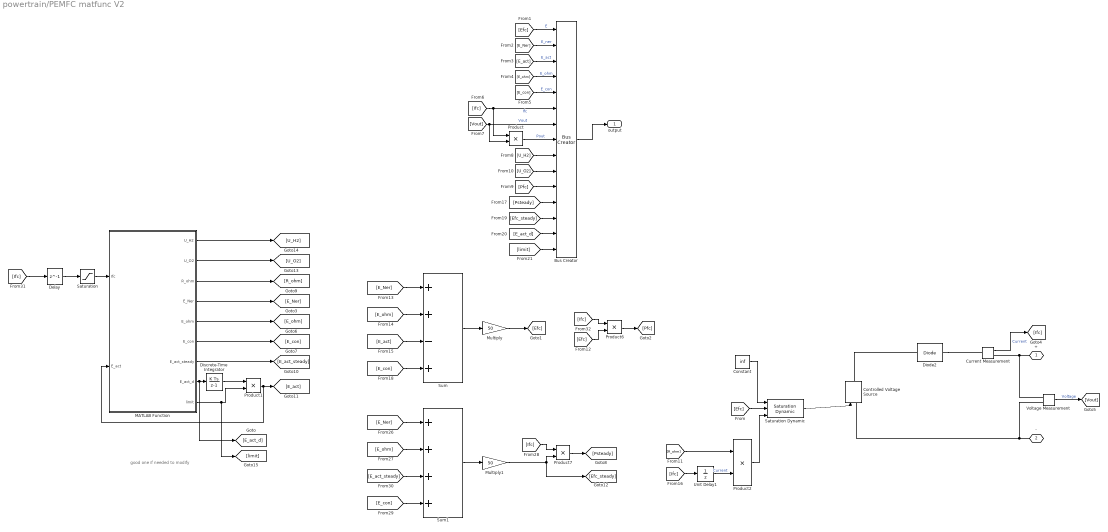
== system powertrain/PEMFC matfunc V2 ==
  note: good one if needed to modify
  Bus Creator : BusCreator  Inputs=15
  Constant : Constant  Value=inf
  Controlled Voltage Source : powerlib/Electrical Sources/Controlled Voltage Source  Initialize=on  Source_Type=AC  Amplitude=0  Phase=0  Frequency=0  Measurements=None
  Current Measurement : powerlib/Measurements/Current Measurement  PhasorSimulation=off  OutputType=Complex  PSBequivalent=0
  Delay : Delay  DelayLength=1
  Diode2 : powerlib/Power Electronics/Diode  Ron=Rohm  Lon=0  Vf=0  IC=0  UseSnubber=off  Rs=1e4  Cs=inf  Measurements=off
  Discrete-Time Integrator : DiscreteIntegrator  SampleTime=-1  ICPrevOutput=DiscIntNeverNeededParam  ICPrevScaledInput=DiscIntNeverNeededParam
  MATLAB Function : MATLAB Function  TreatAsAtomicUnit=on
  Multiply : Gain  Gain=50
  Multiply1 : Gain  Gain=50
  Product{,1..2,6..7} (5 alike) : Product
  Saturation : Saturate  UpperLimit=inf  LowerLimit=0.001
  Saturation Dynamic : simulink/Discontinuities/Saturation Dynamic  OutMin=[]  OutMax=[]  OutDataTypeStr=Inherit: Same as second input  OutDataType=fixdt(1, 16)  OutScaling=2^-10  DoSatur=off
  Sum : Sum  Inputs=++-+
  Sum1 : Sum  Inputs=++++
  Unit Delay1 : UnitDelay  SampleTime=Ts  HasFrameUpgradeWarning=on
  Voltage Measurement : powerlib/Measurements/Voltage Measurement  PhasorSimulation=off  OutputType=Complex  PSBequivalent=0
  + : PMIOPort  Tag=PMCPort  Side=Right
  - : PMIOPort  Tag=PMCPort  Port=2  Side=Right
  output : Outport  VectorParamsAs1DForOutWhenUnconnected=off
  wires:
  [Efc] -> Bus Creator/1  "E"
  [E_Ner] -> Bus Creator/2  "E_ner"
  [E_act] -> Bus Creator/3  "E_act"
  [E_ohm] -> Bus Creator/4  "E_ohm"
  [Ifc] -> Product/1, Bus Creator/6  "Ifc"
  [Vout] -> Product/2, Bus Creator/7  "Vout"
  [E_con] -> Bus Creator/5  "E_con"
  Product/1 -> Bus Creator/8  "Pout"
  Current Measurement/1 -> [Ifc]  "Current"
  Voltage Measurement/1 -> [Vout]  "Voltage"
  [U_H2] -> Bus Creator/9
  [U_O2] -> Bus Creator/10
  Bus Creator/1 -> output/1
  [Ifc] -> Unit Delay1/1
  Unit Delay1/1 -> Product2/2  "Current"
  Product2/1 -> Saturation Dynamic/3
  [R_ohm] -> Product2/1
  Constant/1 -> Saturation Dynamic/1
  Saturation Dynamic/1 -> Controlled Voltage Source/1
  MATLAB Function/3(R_ohm) -> [R_ohm]
  MATLAB Function/7(E_act_steady) -> [E_act_steady]
  MATLAB Function/5(E_ohm) -> [E_ohm]
  Discrete-Time Integrator/1 -> Product1/1
  [Efc] -> Product6/2
  [E_ohm] -> Sum1/2
  Multiply1/1 -> [Efc_steady], Product7/2
  [E_con] -> Sum1/4
  [Ifc] -> Product7/1
  [E_ohm] -> Sum/2
  [E_act] -> Sum/3
  Product6/1 -> [Pfc]
  [E_act_steady] -> Sum1/3
  Sum1/1 -> Multiply1/1
  Sum/1 -> Multiply/1
  MATLAB Function/4(E_Ner) -> [E_Ner]
  [E_con] -> Sum/4
  MATLAB Function/6(E_con) -> [E_con]
  [Ifc] -> Product6/1
  [E_Ner] -> Sum1/1
  [Ifc] -> Delay/1
  Multiply/1 -> [Efc]
  MATLAB Function/8(E_act_d) -> [E_act_d], Discrete-Time Integrator/1
  [E_Ner] -> Sum/1
  [Efc] -> Saturation Dynamic/2
  Product7/1 -> [Psteady]
  [Efc_steady] -> Bus Creator/13
  [Pfc] -> Bus Creator/11
  [Psteady] -> Bus Creator/12
  MATLAB Function/1(U_H2) -> [U_H2]
  MATLAB Function/2(U_O2) -> [U_O2]
  Saturation/1 -> MATLAB Function/1(Ifc)
  Delay/1 -> Saturation/1
  Product1/1 -> MATLAB Function/2(E_act), [E_act]
  MATLAB Function/9(limit) -> [limit], Product1/2
  [E_act_d] -> Bus Creator/14
  [limit] -> Bus Creator/15
  connections:
  -/RConn1 -- Voltage Measurement/LConn2 -- Controlled Voltage Source/LConn1
  +/RConn1 -- Voltage Measurement/LConn1 -- Current Measurement/RConn1
  Diode2/RConn1 -- Current Measurement/LConn1
  Diode2/LConn1 -- Controlled Voltage Source/RConn1

== system powertrain/PEMFC matfunc V3 - multi ==
  note: good one if needed to modify
  Bus Creator : BusCreator  Inputs=15
  Constant : Constant  Value=inf
  Controlled Voltage Source : powerlib/Electrical Sources/Controlled Voltage Source  Initialize=on  Source_Type=AC  Amplitude=0  Phase=0  Frequency=0  Measurements=None
  Current Measurement : powerlib/Measurements/Current Measurement  PhasorSimulation=off  OutputType=Complex  PSBequivalent=0
  Delay : Delay  DelayLength=1
  Diode2 : powerlib/Power Electronics/Diode  Ron=Rohm  Lon=0  Vf=0  IC=0  UseSnubber=off  Rs=1e4  Cs=inf  Measurements=off
  Discrete-Time Integrator : DiscreteIntegrator  SampleTime=-1  ICPrevOutput=DiscIntNeverNeededParam  ICPrevScaledInput=DiscIntNeverNeededParam
  MATLAB Function : MATLAB Function  TreatAsAtomicUnit=on
  Multiply : Gain  Gain=50
  Multiply1 : Gain  Gain=50
  Product{,1..2,6..7} (5 alike) : Product
  Saturation : Saturate  UpperLimit=inf  LowerLimit=0.001
  Saturation Dynamic : simulink/Discontinuities/Saturation Dynamic  OutMin=[]  OutMax=[]  OutDataTypeStr=Inherit: Same as second input  OutDataType=fixdt(1, 16)  OutScaling=2^-10  DoSatur=off
  Sum : Sum  Inputs=++-+
  Sum1 : Sum  Inputs=++++
  Unit Delay1 : UnitDelay  SampleTime=Ts  HasFrameUpgradeWarning=on
  Voltage Measurement : powerlib/Measurements/Voltage Measurement  PhasorSimulation=off  OutputType=Complex  PSBequivalent=0
  + : PMIOPort  Tag=PMCPort  Side=Right
  - : PMIOPort  Tag=PMCPort  Port=2  Side=Right
  output : Outport  VectorParamsAs1DForOutWhenUnconnected=off
  wires:
  [limit] -> Bus Creator/15
  [E_act_d] -> Bus Creator/14
  MATLAB Function/9(limit) -> Product1/2, [limit]
  Product1/1 -> [E_act], MATLAB Function/2(E_act)
  Delay/1 -> Saturation/1
  Saturation/1 -> MATLAB Function/1(Ifc)
  MATLAB Function/2(U_O2) -> [U_O2]
  MATLAB Function/1(U_H2) -> [U_H2]
  [Psteady] -> Bus Creator/12
  [Pfc] -> Bus Creator/11
  [Efc_steady] -> Bus Creator/13
  Product7/1 -> [Psteady]
  [Efc] -> Saturation Dynamic/2
  [E_Ner] -> Sum/1
  MATLAB Function/8(E_act_d) -> Discrete-Time Integrator/1, [E_act_d]
  Multiply/1 -> [Efc]
  [Ifc] -> Delay/1
  [E_Ner] -> Sum1/1
  [Ifc] -> Product6/1
  MATLAB Function/6(E_con) -> [E_con]
  [E_con] -> Sum/4
  MATLAB Function/4(E_Ner) -> [E_Ner]
  Sum/1 -> Multiply/1
  Sum1/1 -> Multiply1/1
  [E_act_steady] -> Sum1/3
  Product6/1 -> [Pfc]
  [E_act] -> Sum/3
  [E_ohm] -> Sum/2
  [Ifc] -> Product7/1
  [E_con] -> Sum1/4
  Multiply1/1 -> Product7/2, [Efc_steady]
  [E_ohm] -> Sum1/2
  [Efc] -> Product6/2
  Discrete-Time Integrator/1 -> Product1/1
  MATLAB Function/5(E_ohm) -> [E_ohm]
  MATLAB Function/7(E_act_steady) -> [E_act_steady]
  MATLAB Function/3(R_ohm) -> [R_ohm]
  Saturation Dynamic/1 -> Controlled Voltage Source/1
  Constant/1 -> Saturation Dynamic/1
  [R_ohm] -> Product2/1
  Product2/1 -> Saturation Dynamic/3
  Unit Delay1/1 -> Product2/2  "Current"
  [Ifc] -> Unit Delay1/1
  Bus Creator/1 -> output/1
  [U_O2] -> Bus Creator/10
  [U_H2] -> Bus Creator/9
  Voltage Measurement/1 -> [Vout]  "Voltage"
  Current Measurement/1 -> [Ifc]  "Current"
  Product/1 -> Bus Creator/8  "Pout"
  [E_con] -> Bus Creator/5  "E_con"
  [Vout] -> Bus Creator/7, Product/2  "Vout"
  [Ifc] -> Bus Creator/6, Product/1  "Ifc"
  [E_ohm] -> Bus Creator/4  "E_ohm"
  [E_act] -> Bus Creator/3  "E_act"
  [E_Ner] -> Bus Creator/2  "E_ner"
  [Efc] -> Bus Creator/1  "E"
  connections:
  Diode2/LConn1 -- Controlled Voltage Source/RConn1
  Diode2/RConn1 -- Current Measurement/LConn1
  Current Measurement/RConn1 -- Voltage Measurement/LConn1 -- +/RConn1
  Controlled Voltage Source/LConn1 -- Voltage Measurement/LConn2 -- -/RConn1

== system powertrain/PV MODULE1 ==
  TempCell_C : Inport
  Irradiance : Inport  Port=2
  Bus Creator : BusCreator  Inputs=4
  Constant : Constant  Value=Ncell
  Constant1 : Constant  Value=Voc
  Constant11 : Constant  Value=df
  Constant12 : Constant  Value=Rsh
  Constant13 : Constant  Value=Rs
  Constant14 : Constant  Value=Npar
  Constant15 : Constant  Value=Nser
  Constant2 : Constant  Value=Isc
  Constant3 : Constant  Value=Vmpp
  Constant4 : Constant  Value=Impp
  Constant5 : Constant  Value=alpha
  Constant6 : Constant  Value=beta_Voc
  Constant7 : Constant  Value=Isc
  Constant8 : Constant  Value=I0
  Controlled Current Source : powerlib/Electrical Sources/Controlled Current Source  Initialize=on  Source_Type=AC  Amplitude=0  Phase=0  Frequency=0  Measurements=None
  Current Measurement : powerlib/Measurements/Current Measurement  PhasorSimulation=off  OutputType=Complex  PSBequivalent=0
  Diode : powerlib/Power Electronics/Diode  Ron=0.001  Lon=0  Vf=0.8  IC=0  UseSnubber=0  Rs=500  Cs=250e-9  Measurements=off
  PV_function : MATLAB Function  TreatAsAtomicUnit=on
  Product : Product
  Unit Delay1 : UnitDelay  SampleTime=Ts  HasFrameUpgradeWarning=on
  Unit Delay4 : UnitDelay  SampleTime=Ts  HasFrameUpgradeWarning=on
  Voltage Measurement : powerlib/Measurements/Voltage Measurement  PhasorSimulation=off  OutputType=Complex  PSBequivalent=0
  + : PMIOPort  Side=Right
  - : PMIOPort  Port=2  Side=Right
  data : Outport
  wires:
  [V_PV] -> Unit Delay1/1
  [I_PV] -> Unit Delay4/1
  Unit Delay4/1 -> PV_function/13(I_PV)
  Unit Delay1/1 -> PV_function/12(V_PV)
  Bus Creator/1 -> data/1
  [V_PV] -> Bus Creator/3  "V_PV"
  [I_PV] -> Bus Creator/2  "I_PV"
  [P_PV] -> Bus Creator/1  "P_PV"
  Product/1 -> [P_PV]
  [I_PV] -> Product/2
  [V_PV] -> Product/1
  Current Measurement/1 -> [I_PV]
  Voltage Measurement/1 -> [V_PV]
  Constant12/1 -> PV_function/15(Rp)
  Constant8/1 -> PV_function/11(I_0)
  Constant13/1 -> PV_function/16(Rs)
  Constant11/1 -> PV_function/14(a)
  PV_function/1(ID) -> Controlled Current Source/1
  Constant2/1 -> PV_function/5(Isc)
  Constant4/1 -> PV_function/7(Imp)
  Constant5/1 -> PV_function/8(alpha)
  Constant7/1 -> PV_function/10(IPH_STC)
  TempCell_C/1 -> [TC]
  Constant6/1 -> PV_function/9(beta)
  Constant1/1 -> PV_function/4(Voc)
  Irradiance/1 -> PV_function/2(Irradiance)
  Constant14/1 -> PV_function/17(para_string)
  Constant15/1 -> PV_function/18(serie_string)
  Constant3/1 -> PV_function/6(Vmp)
  Constant/1 -> PV_function/3(Ncell)
  [TC] -> Bus Creator/4  "Temperature (deg C)"
  [TC] -> PV_function/1(TempCell_C)
  connections:
  Diode/LConn1 -- Controlled Current Source/RConn1
  Current Measurement/LConn1 -- Diode/RConn1
  Voltage Measurement/LConn1 -- +/RConn1 -- Current Measurement/RConn1
  Controlled Current Source/LConn1 -- Voltage Measurement/LConn2 -- -/RConn1

== system powertrain/Subsystem ==
  In1 : Inport
  Constant : Subsystem  VariantControl=Constant
  Model1 : Subsystem  VariantControl=Model1
  Step : Subsystem  VariantControl=Step
  Out1 : Outport

== system powertrain/EMS/Management Variant ==
  PV : Inport
  FC : Inport  Port=2
  SC : Inport  Port=3
  BATT : Inport  Port=4
  LOAD : Inport  Port=5
  ANFIS-ECMS : Subsystem  VariantControl=ANFIS-ECMS
  Constant : Subsystem  VariantControl=CONSTANT
  D-ECMS : Subsystem  VariantControl=D-ECMS
  ECAEMS : Subsystem  VariantControl=ECAEMS
  ECMS : Subsystem  VariantControl=ECMS
  EEMS : Subsystem  VariantControl=EEMS
  FUZZY : Subsystem  VariantControl=FUZZY
  MPC-1 : Subsystem  VariantControl=MPC-1
  PI : Subsystem  VariantControl=PI
  SMC : Subsystem  VariantControl=SMC
  Vbatt_conv : Outport
  Ibatt_conv : Outport  Port=2
  batt converter mode : Outport  Port=3
  I/O batt conv : Outport  Port=4
  Vfc_conv : Outport  Port=5
  Ifc_conv : Outport  Port=6
  I/O fc conv : Outport  Port=7
  Vpv_conv : Outport  Port=8
  Ipv_conv : Outport  Port=9
  I/O pv conv : Outport  Port=10
  PV control mode : Outport  Port=11

== system powertrain/Load1/Constant ==
  In1 : Inport
  Constant : Constant  Value=CstVal
  Out1 : Outport
  wires:
  Constant/1 -> Out1/1
